simulink model "simulateDBPSK_pulseShaping"  (R2017a)
settings: Solver=VariableStepAuto  StartTime=0.0  StopTime=10  RelTol=1e-3
InitFcn:
  | fs = 60e3;
libraries: commdigbbndpm3 x2, commfilt2 x2, commchan3 x1, commrandsrc3 x1, commsink2 x1, commrflib2 x1
settings Model: Creator=prust  LastModifiedBy=prust

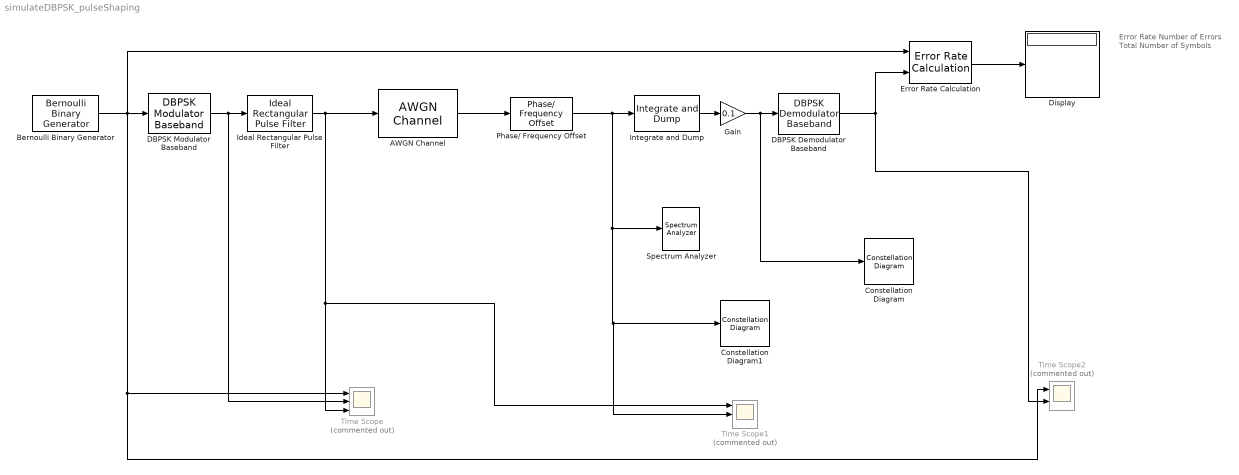
== system simulateDBPSK_pulseShaping ==
  note: Error Rate
      |
      | Number of Errors
      |
      | Total Number of Symbols
  AWGN Channel : commchan3/AWGN Channel  InputProcessing=Columns as channels (frame based)  seed=67  noiseMode="Signal to noise ratio  (Eb/No)"  EbNodB=9  EsNodB=10  SNRdB=10  bitsPerSym=1  Ps=1  Tsym=1/fs  variance=1
  Bernoulli Binary Generator : commrandsrc3/Bernoulli Binary Generator  ProbabilityOfZero=0.5  SeedSource=Auto  Seed=0  SampleTime=1/fs  SamplesPerFrame=1000  OutputDataType=double  SimulateUsing=Interpreted execution
  Constellation Diagram : ConstellationDiagram
  Constellation Diagram1 : ConstellationDiagram
  DBPSK Demodulator Baseband : commdigbbndpm3/DBPSK Demodulator Baseband  Ph=0  outDtype=Inherit via internal rule
      settings: SourceProductName=Communications System Toolbox  SourceProductBaseCode=CM
  DBPSK Modulator Baseband : commdigbbndpm3/DBPSK Modulator Baseband  Ph=0  outDtype=double
      settings: SourceProductName=Communications System Toolbox  SourceProductBaseCode=CM
  Display : Display
  Error Rate Calculation : commsink2/Error Rate Calculation  N=0  st_delay=0  cp_mode=Entire frame  subframe=[]  PMode=Port  WsName=ErrorVec  RsMode2=off  stop=off  numErr=100  maxBits=1e6
  Gain : Gain  Gain=0.1
  Ideal Rectangular Pulse Filter : commfilt2/Ideal Rectangular Pulse Filter  pulseLen=10  pulseDelay=0  InputProcessing=Columns as channels (frame based)  RateOptions=Enforce single-rate processing  sampMode=Mute  normCheck=off  normMode=Sum of samples  filterGain=1  saveAsFlag=0  roundingMode=Floor  overflowMode=off  firstCoeffDataTypeStr=Inherit: Same word length as input  firstCoeffMin=[]  firstCoeffMax=[]  firstCoeffLastDataTypeStr=Inherit: Same word length as input  outputDataTypeStr=Inherit: Same as accumulator  outputMin=[]  outputMax=[]  outputLastDataTypeStr=Inherit: Same as accumulator
      settings: SourceProductName=Communications System Toolbox  SourceProductBaseCode=CM
  Integrate and Dump : commfilt2/Integrate and Dump  obssamples=10  offsetsamples=0  nodump=off  roundingMode=Floor  overflowMode=off  outputDataTypeStr=Inherit: Same as accumulator  outputLastDataTypeStr=Inherit: Same as accumulator
      settings: SourceProductName=Communications System Toolbox
  Phase/ Frequency Offset : commrflib2/Phase// Frequency Offset  phaseOffset=0  freqPort=off  freqOffset=100
      settings: SourceProductName=Communications System Toolbox
  Spectrum Analyzer : SpectrumAnalyzer
  Time Scope : Scope  Commented=on  NumInputPorts=3
  Time Scope1 : Scope  Commented=on  NumInputPorts=3
  Time Scope2 : Scope  Commented=on  NumInputPorts=2
  wires:
  Bernoulli Binary Generator/1 -> Time Scope2/1, Time Scope/1, DBPSK Modulator Baseband/1, Error Rate Calculation/1
  DBPSK Modulator Baseband/1 -> Time Scope/2, Ideal Rectangular Pulse Filter/1
  AWGN Channel/1 -> Phase/ Frequency Offset/1
  DBPSK Demodulator Baseband/1 -> Time Scope2/2, Error Rate Calculation/2
  Error Rate Calculation/1 -> Display/1
  Integrate and Dump/1 -> Gain/1
  Ideal Rectangular Pulse Filter/1 -> AWGN Channel/1, Time Scope1/1, Time Scope/3
  Phase/ Frequency Offset/1 -> Spectrum Analyzer/1, Time Scope1/2, Constellation Diagram1/1, Integrate and Dump/1
  Gain/1 -> DBPSK Demodulator Baseband/1, Constellation Diagram/1
